simulink model "MatlabFunDemo"  (R2014a)
settings: Solver=ode45  StartTime=0.0  StopTime=10.0  RelTol=1e-3
settings Model: Creator=lgw  LastModifiedBy=李广文

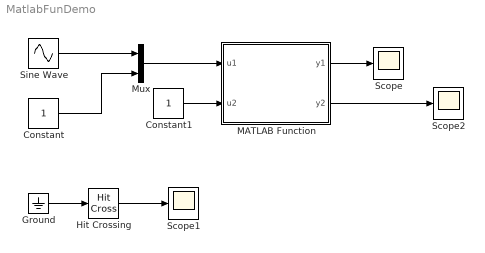
== system MatlabFunDemo ==
  Constant : Constant
  Constant1 : Constant
  Ground : Ground
  Hit Crossing : HitCross
  MATLAB Function : MATLAB Function  TreatAsAtomicUnit=on
  Mux : Mux  Inputs=2
  Scope : Scope
  Scope1 : Scope
  Scope2 : Scope
      settings: SaveName=ScopeData2
  Sine Wave : Sin
  wires:
  MATLAB Function/1(y1) -> Scope/1
  Sine Wave/1 -> Mux/1
  Constant/1 -> Mux/2
  Mux/1 -> MATLAB Function/1(u1)
  Hit Crossing/1 -> Scope1/1
  Constant1/1 -> MATLAB Function/2(u2)
  MATLAB Function/2(y2) -> Scope2/1
  Ground/1 -> Hit Crossing/1

== matlab function MatlabFunDemo/MATLAB Function ==
  data: u1 input; y1 output; u2 input; y2 output
function [y1,y2]= MyFun(u1,u2)
%#codegen
if u1(1)>0
    y1 = u1(1)+u1(2);
else
     y1 = u1(1)-u1(2);
end
% A=cell(2);
% A{1}=u2;
% y2=A{1};
y2=u2;
